simulink model "Pos_c_CodeTesting_pract"  (R2022a)
settings: Solver=VariableStepAuto  StartTime=0.0  StopTime=20  RelTol=1e-3
undefined symbols (not defined in the file or in its folder): A_0, A_0k, d, F_0, F_0k, g, Gi_s, Gp_s, ktd_s, m, M, P_0, P_0k, Ts
settings Model: Creator=DELL  LastModifiedBy=DELL

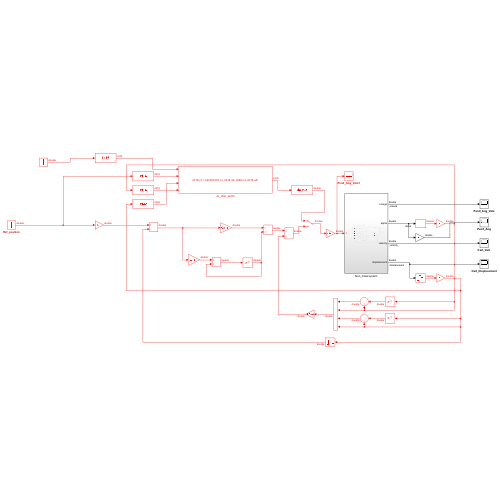
[thumbnail: Simulink's stored preview of the top-level diagram]
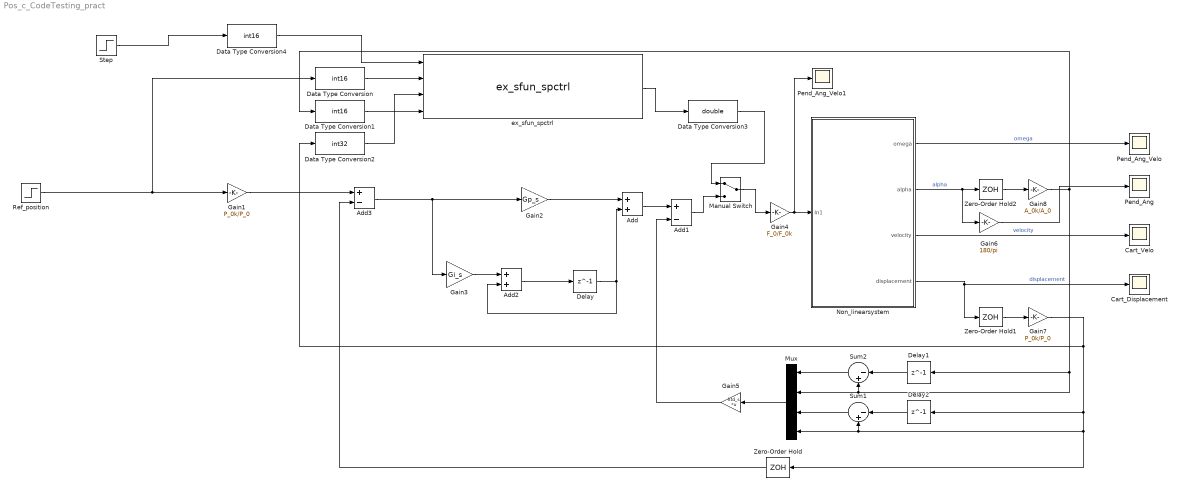
== system Pos_c_CodeTesting_pract ==
  Add : Sum
  Add1 : Sum  Inputs=+-
  Add2 : Sum
  Add3 : Sum  Inputs=+-
  Cart_Displacement : Scope
  Cart_Velo : Scope
  Data Type Conversion : DataTypeConversion  OutDataTypeStr=int16  SaturateOnIntegerOverflow=off  RndMeth=Floor
  Data Type Conversion1 : DataTypeConversion  OutDataTypeStr=int16  SaturateOnIntegerOverflow=off  RndMeth=Floor
  Data Type Conversion2 : DataTypeConversion  OutDataTypeStr=int32  SaturateOnIntegerOverflow=off  RndMeth=Floor
  Data Type Conversion3 : DataTypeConversion  OutDataTypeStr=double  SaturateOnIntegerOverflow=off  RndMeth=Floor
  Data Type Conversion4 : DataTypeConversion  OutDataTypeStr=int16  SaturateOnIntegerOverflow=off  RndMeth=Floor
  Delay : Delay  DelayLength=1  SampleTime=Ts
  Delay1 : Delay  DelayLength=1  SampleTime=Ts
  Delay2 : Delay  DelayLength=1  SampleTime=Ts
  Gain1 : Gain  Gain=P_0k/P_0
  Gain2 : Gain  Gain=Gp_s
  Gain3 : Gain  Gain=Gi_s
  Gain4 : Gain  Gain=F_0/F_0k
  Gain5 : Gain  Gain=ktd_s  Multiplication=Matrix(K*u) (u vector)
  Gain6 : Gain  Gain=180/pi
  Gain7 : Gain  Gain=P_0k/P_0
  Gain8 : Gain  Gain=A_0k/A_0
  Manual Switch : ManualSwitch
  Mux : Mux
  Non_linearsystem : Subsystem
  Pend_Ang : Scope
  Pend_Ang_Velo : Scope
  Pend_Ang_Velo1 : Scope
  Ref_position : Step  SampleTime=Ts
  Step : Step  Time=2*Ts  Before=1  After=0  SampleTime=Ts
  Sum1 : Sum  Inputs=|-+
  Sum2 : Sum  Inputs=|-+
  Zero-Order Hold : ZeroOrderHold  SampleTime=Ts
  Zero-Order Hold1 : ZeroOrderHold  SampleTime=Ts
  Zero-Order Hold2 : ZeroOrderHold  SampleTime=Ts
  ex_sfun_spctrl : S-Function  FunctionName=ex_sfun_spctrl  SFunctionDeploymentMode=off  EnableBusSupport=off  mask(Legacy Function){SFunctionSpec=int16 y1 = spctrl(int16 u1, int16 u2, int32 u3, int16 u4), ShowSpec=on}
      mask prompts: ShowSpec "Display function specification"
      mask help:
      | This block allows you to call the legacy functions specified by the following Legacy Code Tool definition:
      | def.SFunctionName = 'ex_sfun_spctrl';
      | def.OutputFcnSpec = 'int16 y1 = spctrl(int16 u1, int16 u2, int32 u3, int16 u4)';
      | def.HeaderFiles = {'xil_types.h', 'Fixedpt_Position_Control.h'};
      mask Help: <p>This block was generated automatically by the Legacy Code Tool. For detailed help on this tool, call<a href="matlab:legacy_code('help')"> legacy_code('help')</a>.</p>
      mask Callback ShowSpec:
      | if strcmp(get_param(gcbh, 'ShowSpec'), 'on')
      |   set_param(gcbh, 'MaskDisplay', sprintf('fprintf(''%s'');', get_param(gcbh, 'SFunctionSpec')));
      | else
      |   set_param(gcbh, 'MaskDisplay', sprintf('fprintf(''%s'');', get_param(gcbh, 'FunctionName')));
      | end
      mask Display: fprintf('int16 y1 = spctrl(int16 u1, int16 u2, int32 u3, int16 u4)');
  wires:
  Gain2/1 -> Add/1
  Delay/1 -> Add/2, Add2/2
  Gain5/1 -> Add1/2
  Add/1 -> Add1/1
  Sum1/1 -> Mux/3
  Gain8/1 -> Delay1/1, Mux/2, Sum2/2, Data Type Conversion1/1
  Delay1/1 -> Sum2/1
  Mux/1 -> Gain5/1
  Add3/1 -> Gain3/1, Gain2/1
  Add2/1 -> Delay/1
  Sum2/1 -> Mux/1
  Zero-Order Hold/1 -> Add3/2
  Delay2/1 -> Sum1/1
  Non_linearsystem/4(displacement) -> Cart_Displacement/1, Zero-Order Hold1/1  "displacement"
  Zero-Order Hold2/1 -> Gain8/1
  Gain4/1 -> Pend_Ang_Velo1/1, Non_linearsystem/1(In1)
  Non_linearsystem/2(alpha) -> Zero-Order Hold2/1, Gain6/1  "alpha"
  Zero-Order Hold1/1 -> Gain7/1
  Gain3/1 -> Add2/1
  Manual Switch/1 -> Gain4/1
  Data Type Conversion3/1 -> Manual Switch/1
  Add1/1 -> Manual Switch/2
  Non_linearsystem/1(omega) -> Pend_Ang_Velo/1  "omega"
  Non_linearsystem/3(velocity) -> Cart_Velo/1  "velocity"
  Gain6/1 -> Pend_Ang/1
  Gain7/1 -> Data Type Conversion2/1, Mux/4, Sum1/2, Zero-Order Hold/1, Delay2/1
  Gain1/1 -> Add3/1
  ex_sfun_spctrl/1 -> Data Type Conversion3/1
  Ref_position/1 -> Data Type Conversion/1, Gain1/1
  Step/1 -> Data Type Conversion4/1
  Data Type Conversion/1 -> ex_sfun_spctrl/2
  Data Type Conversion1/1 -> ex_sfun_spctrl/4
  Data Type Conversion2/1 -> ex_sfun_spctrl/3
  Data Type Conversion4/1 -> ex_sfun_spctrl/1

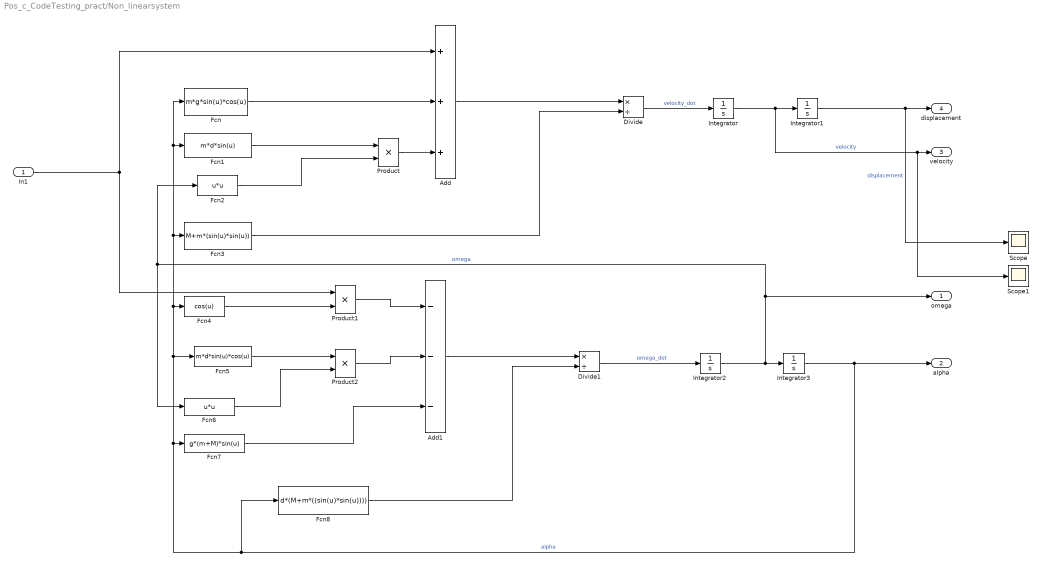
== system Pos_c_CodeTesting_pract/Non_linearsystem ==
  In1 : Inport
  Add : Sum  Inputs=+++
  Add1 : Sum  Inputs=---
  Divide : Product  Inputs=*/
  Divide1 : Product  Inputs=*/
  Fcn : Fcn  Expr=m*g*sin(u)*cos(u)
  Fcn1 : Fcn  Expr=m*d*sin(u)
  Fcn2 : Fcn  Expr=u*u
  Fcn3 : Fcn  Expr=M+m*(sin(u)*sin(u))
  Fcn4 : Fcn  Expr=cos(u)
  Fcn5 : Fcn  Expr=m*d*sin(u)*cos(u)
  Fcn6 : Fcn  Expr=u*u
  Fcn7 : Fcn  Expr=g*(m+M)*sin(u)
  Fcn8 : Fcn  Expr=d*(M+m*((sin(u)*sin(u))))
  Integrator{,1..3} (4 alike) : Integrator
  Product : Product
  Product1 : Product
  Product2 : Product
  Scope : Scope
  Scope1 : Scope
  omega : Outport  VectorParamsAs1DForOutWhenUnconnected=off
  alpha : Outport  Port=2  VectorParamsAs1DForOutWhenUnconnected=off
  velocity : Outport  Port=3  VectorParamsAs1DForOutWhenUnconnected=off
  displacement : Outport  Port=4  VectorParamsAs1DForOutWhenUnconnected=off
  wires:
  Add/1 -> Divide/1
  Integrator2/1 -> Integrator3/1, omega/1, Fcn2/1, Fcn6/1  "omega"
  Fcn1/1 -> Product/1
  Integrator1/1 -> Scope/1, displacement/1  "displacement"
  Fcn6/1 -> Product2/2
  Product/1 -> Add/3
  Fcn2/1 -> Product/2
  Fcn4/1 -> Product1/2
  Fcn/1 -> Add/2
  Integrator3/1 -> alpha/1, Fcn8/1, Fcn7/1, Fcn5/1, Fcn4/1, Fcn/1, Fcn1/1, Fcn3/1  "alpha"
  Divide/1 -> Integrator/1  "velocity_dot"
  Fcn3/1 -> Divide/2
  Product2/1 -> Add1/2
  Add1/1 -> Divide1/1
  Fcn5/1 -> Product2/1
  Product1/1 -> Add1/1
  Fcn8/1 -> Divide1/2
  Fcn7/1 -> Add1/3
  In1/1 -> Add/1, Product1/1
  Integrator/1 -> Integrator1/1, Scope1/1, velocity/1  "velocity"
  Divide1/1 -> Integrator2/1  "omega_dot"
